simulink model "PD_SeguimientoTrayectoria"  (R2020b)
settings: Solver=VariableStepAuto  StartTime=0.0  StopTime=10  RelTol=1e-3
libraries: fl_lib x5, nesl_utility x3, ee_lib x1
settings Model: Creator=petir  LastModifiedBy=petir
settings SolverCC: AlgebraicLoopSolver=LineSearch

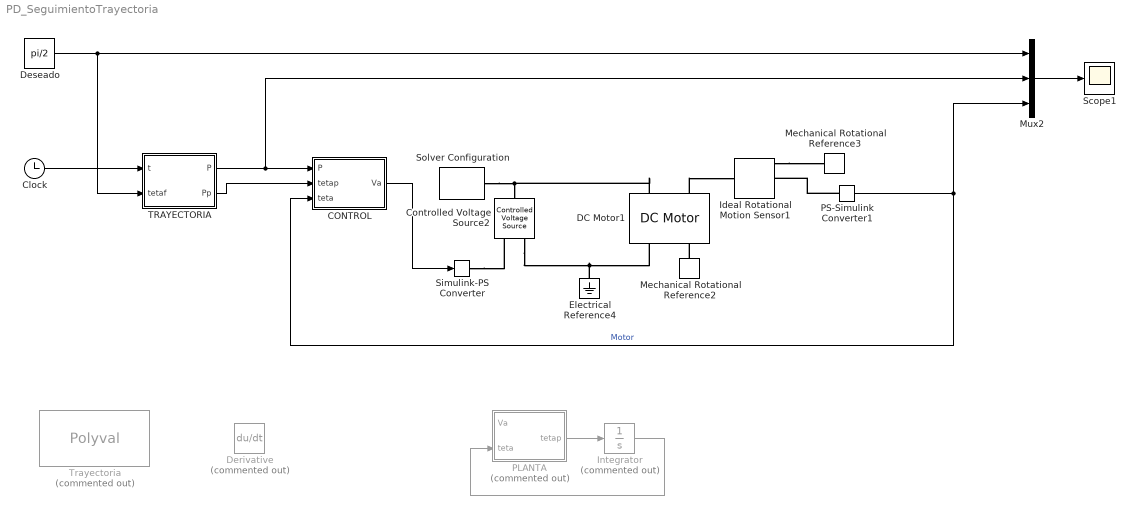
== system PD_SeguimientoTrayectoria ==
  CONTROL : MATLAB Function  TreatAsAtomicUnit=on
  Clock : Clock
  Controlled Voltage Source2 : fl_lib/Electrical/Electrical Sources/Controlled Voltage Source
  DC Motor1 : ee_lib/Electromechanical/Brushed Motors/DC Motor  field_option=ee.enum.field_option.pm  Rf=100 Ohm  Lf=1 H  Laf=0.15 H  If0=0 A  parameterization=ee.enum.dcparam_option.circuit_param  Ra=8.3 Ohm  La=1.51e-3 H  emf_or_torque=ee.enum.emf_or_torque.ki  Kv=0.0879 V/(rad/s)  Ki=0.0879 N*m/A  T_stall=0.24e-3 N*m  w_max=19100 rpm  w_rated=15000 rpm  P_rated=0.08 W  V_rated=1.5 V  J=80.7e-6 kg*m^2  lam_param=ee.enum.lam_param.damping  lam=14.41e-6 N*m/(rad/s)  i_noload=0 A  V_i_noload=1.5 V  speed0=0 rpm  enable_fault_armature=ee.enum.faults.faultEnable.no  rev_faulted=1 / 3  G_faulted_armature=1e-5 S  fault_trigger_armature=ee.enum.faults.faultTrigger.temporal  t_fault_armature=1 s  max_permissible_current_armature=inf A  t_fail_on_current_armature=1 s  enable_fault_field=ee.enum.faults.faultEnable.no  G_faulted_field=1e-5 S  fault_trigger_field=ee.enum.faults.faultTrigger.temporal  t_fault_field=1 s  max_permissible_current_field=inf A  t_fail_on_current_field=1 s  fault_action=ee.enum.faults.faultAction.none  alpha=3.93e-3 1/K  Tmeas=25 degC  thermal_mass=100 J/K  initial_temperature=25 degC
  Derivative : Derivative  Commented=on
  Deseado : Constant  Value=pi/2  VectorParams1D=off
  Electrical Reference4 : fl_lib/Electrical/Electrical Elements/Electrical Reference
  Ideal Rotational Motion Sensor1 : fl_lib/Mechanical/Mechanical Sensors/Ideal Rotational Motion Sensor  wrap_angle=simscape.enum.onoff.off  offset=0 rad
  Integrator : Integrator  Commented=on
  Mechanical Rotational Reference2 : fl_lib/Mechanical/Rotational Elements/Mechanical Rotational Reference
  Mechanical Rotational Reference3 : fl_lib/Mechanical/Rotational Elements/Mechanical Rotational Reference
  Mux2 : Mux  Inputs=3
  PLANTA : MATLAB Function  Commented=on  TreatAsAtomicUnit=on
  PS-Simulink Converter1 : nesl_utility/PS-Simulink Converter  PhysicalDomain=network_engine_domain  SubClassName=ps_output  LeftPortType=input  RightPortType=output  PseudoPeriodic=off  Frequencies=[]  Unit=inherit  AffineConversion=off
  Scope1 : Scope
  Simulink-PS Converter : nesl_utility/Simulink-PS Converter  PhysicalDomain=network_engine_domain  SubClassName=ps_input  LeftPortType=input  RightPortType=output  PseudoPeriodic=off  Frequencies=[]  NoiseDistribution=none  NoiseParameters=[]  Unit=1  AffineConversion=off  FilteringAndDerivatives=provide  SimscapeFilterOrder=1  InputFilterTimeConstant=0.001  UdotUserProvided=0
  Solver Configuration : nesl_utility/Solver Configuration  PhysicalDomain=network_engine_domain  SubClassName=solver  LeftPortType=input  RightPortType=generic  Tones=[]  Harmonics=[]  SimulateNoise=off  Profile=off  UseLocalSampling=off  EnableSwitchedLinearOptims=on  FrequencyDomain=off  UseCCode=off  RelTol=0.001  AbsTol=1e-06  MinStep=1e-09  ToWorkspace=off  RevertToSquareIcSolve=off  NumHomotopyIterations=100  PhasorMode=off  PhasorModeNumHarmonics=1  DoDC=off  ResidualTolerance=1e-09  UseLocalSolver=off  LocalSolverChoice=NE_BACKWARD_EULER_ADVANCER  LocalSolverSampleTime=0.001  DoFixedCost=off  MaxNonlinIter=3  MaxModeIter=2  ComputeImpulses=off  ImpulseIterations=2  LinearAlgebra=auto  EquationFormulation=NE_TIME_EF  DelaysMemoryBudget=1024  AutomaticFiltering=on  FilteringTimeConstant=0.001  PartitionStorageMethod=AS_NEEDED  PartitionMemoryBudget=1024  PartitionMethod=ROBUST
  TRAYECTORIA : MATLAB Function  TreatAsAtomicUnit=on
  Trayectoria : Polyval  Commented=on  Coefs=[-2*40/1000 3*40/100 0 0]
  wires:
  PLANTA/1(tetap) -> Integrator/1
  PS-Simulink Converter1/1 -> Mux2/3, CONTROL/3(teta)  "Motor"
  Mux2/1 -> Scope1/1
  Clock/1 -> TRAYECTORIA/1(t)
  Deseado/1 -> TRAYECTORIA/2(tetaf), Mux2/1
  Integrator/1 -> PLANTA/2(teta)
  TRAYECTORIA/1(P) -> Mux2/2, CONTROL/1(P)
  TRAYECTORIA/2(Pp) -> CONTROL/2(tetap)
  CONTROL/1(Va) -> Simulink-PS Converter/1
  connections:
  Controlled Voltage Source2/RConn2 -- DC Motor1/RConn1 -- Electrical Reference4/LConn1
  DC Motor1/LConn1 -- Solver Configuration/RConn1 -- Controlled Voltage Source2/LConn1
  DC Motor1/LConn2 -- Ideal Rotational Motion Sensor1/LConn1
  Ideal Rotational Motion Sensor1/RConn1 -- Mechanical Rotational Reference3/LConn1
  PS-Simulink Converter1/LConn1 -- Ideal Rotational Motion Sensor1/RConn2
  Mechanical Rotational Reference2/LConn1 -- DC Motor1/RConn2
  Simulink-PS Converter/RConn1 -- Controlled Voltage Source2/RConn1

== matlab function PD_SeguimientoTrayectoria/CONTROL ==
  data: P input; tetap input; teta input; Va output
function Va = fcn(P, tetap, teta)
% Parametros
Ra = 8.3;
Ke = 0.0879;
Ki = 0.0879;
J = 80.7e-6;
B = 14.41e-6;

tetad = P;

Kp = 25;
Kd = 2;

Vaux = Kp * (tetad - teta) - Kd * tetap;
Va = J * Ra / Ki * (Vaux + Ki * Ke / (J * Ra) * teta + B / J * teta);

== matlab function PD_SeguimientoTrayectoria/PLANTA ==
  data: Va input; tetap output; teta input
% function tetapp = fcn(Va, tetap)
function tetap = fcn(Va, teta)
% Parámetros
Ra = 8.3;
Ke = 0.0879;
Ki = 0.0879;
J = 80.7e-6;
B = 14.41e-6;
TL = 0.1*0;

% Ra = 10.3;
% Ke = 0.0113;
% Ki = 0.0113;
% J = 1.7e-6;
% B = 3.41e-6;
% TL = 0.1*0;


% tetapp = Ki / (J * Ra) * Va - Ki * Ke / (J * Ra) * tetap - B / J * tetap - 1 / J * TL;
tetap = (Ki / (J * Ra)) * Va - (Ki * Ke / (J * Ra)) * teta - (B / J) * teta - 1 / J * TL;

== matlab function PD_SeguimientoTrayectoria/TRAYECTORIA ==
  data: t input; P output; Pp output; tetaf input
function [P, Pp] = fcn(t, tetaf)
% Parametros
teta0 = 0;
tetaf = tetaf;
tetap0 = 0;
tetapf = 0;
% Tiempo de simulación
tf = 10;

P = teta0 + tetap0 * t + (3/tf^2) * (tetaf - teta0) * t^2 - (2/tf^3) * (tetaf - teta0) * t^3;
Pp = teta0 + (6/tf^2) * (tetaf - teta0) * t - (6 / tf^3) * (tetaf - teta0) * t^2;
